simulink model "mass_sim_HW_04"  (R2018a)
settings: Solver=ode45  StartTime=0.0  StopTime=50  MaxStep=1  RelTol=1e-3
InitFcn:
  | mass_spring_damper_param
undefined symbols (not defined in the file or in its folder): mass_spring_damper_animation
settings Model: Creator=canla  LastModifiedBy=canla
settings OptimizationCC: LifeSpan=inf

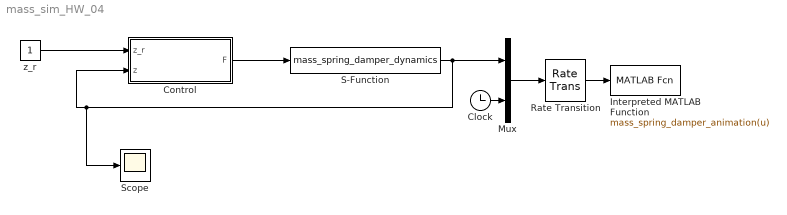
== system mass_sim_HW_04 ==
  Clock : Clock
  Control : Subsystem
  Interpreted MATLAB Function : MATLABFcn  MATLABFcn=mass_spring_damper_animation(u)  OutputDimensions=0
  Mux : Mux  Inputs=2
  Rate Transition : RateTransition  OutPortSampleTime=P.t_plot
  S-Function : S-Function  FunctionName=mass_spring_damper_dynamics  Parameters=P  SFunctionDeploymentMode=off  EnableBusSupport=off
  Scope : Scope
  z_r : Constant
  wires:
  z_r/1 -> Control/1(z_r)
  Control/1(F) -> S-Function/1
  S-Function/1 -> Scope/1, Control/2(z), Mux/1
  Clock/1 -> Mux/2
  Mux/1 -> Rate Transition/1
  Rate Transition/1 -> Interpreted MATLAB Function/1

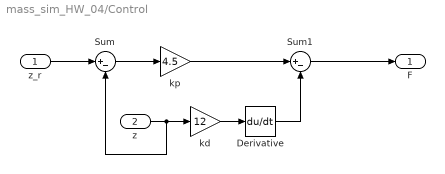
== system mass_sim_HW_04/Control ==
  z_r : Inport
  z : Inport  Port=2
  Derivative : Derivative
  Sum : Sum  Inputs=|+-
  Sum1 : Sum  Inputs=|+-
  kd : Gain  Gain=12
  kp : Gain  Gain=4.5
  F : Outport
  wires:
  z_r/1 -> Sum/1
  z/1 -> Sum/2, kd/1
  Sum/1 -> kp/1
  kp/1 -> Sum1/1
  Sum1/1 -> F/1
  kd/1 -> Derivative/1
  Derivative/1 -> Sum1/2
